simulink model "Homework4_P1"  (R2023b)
settings: Solver=FixedStepDiscrete  StartTime=0.0  StopTime=1  FixedStep=0.002  RelTol=1e-3  EnableMultiTasking=on
values from neighbouring files (symbols this model uses):
  Beta = [B_0 ; B_1 ; B_2 ; B_3]    [Homework4.m]
  phi = 45    [Homework4.m]
  psi = 60    [Homework4.m]
  theta = 30    [Homework4.m]
undefined symbols (not defined in the file or in its folder): a, alpha
settings Model: ExtModeTrigDuration=10000  Creator=jtmil  LastModifiedBy=jtmil
settings SolverCC: AlgebraicLoopSolver=TrustRegion  PositivePriorityOrder=on
settings DataIOCC: ReturnWorkspaceOutputs=off
settings OptimizationCC: LifeSpan=inf
settings DebuggingCC: UnconnectedInputMsg=warning  UnconnectedOutputMsg=warning  UnconnectedLineMsg=warning  ArithmeticOperatorsInVariantConditions=warning
settings ModelReferenceCC: EnableRefExpFcnMdlSchedulingChecks=on
settings SFSimCC: SimUseLocalCustomCode=off  CustomCodeUndefinedFunction=UseInterfaceOnly
settings RTWCC: Description=QUARC Win64 Target  SystemTargetFile=quarc_win64.tlc  TemplateMakefile=quarc_default_tmf  RTWUseLocalCustomCode=off
settings CodeAppCC: StateflowObjectComments=on
settings STFCustomTargetCC: TargetPreCompLibLocation=C:\PROGRA~3\QUARC\lib\2016a\win64\release  ConcurrentExecutionCompliant=on  GRTInterface=on  SystemTargetFile=quarc_win64.tlc
settings GRTTargetCC: TargetPreCompLibLocation=C:\PROGRA~3\QUARC\lib\2016a\win64\release  ParMdlRefBuildCompliant=off  CompOptLevelCompliant=off  CombineOutputUpdateFcns=off  MatFileLogging=off  CPPClassGenCompliant=off  GRTInterface=on  UseToolchainInfoCompliant=off  ExtMode=on  ExtModeMexFile=quarc_comm
settings ConfigComp: CovMetricSettings=dswe

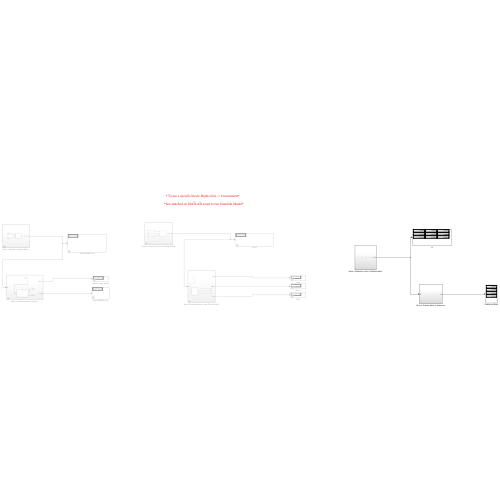
[thumbnail: Simulink's stored preview of the top-level diagram]
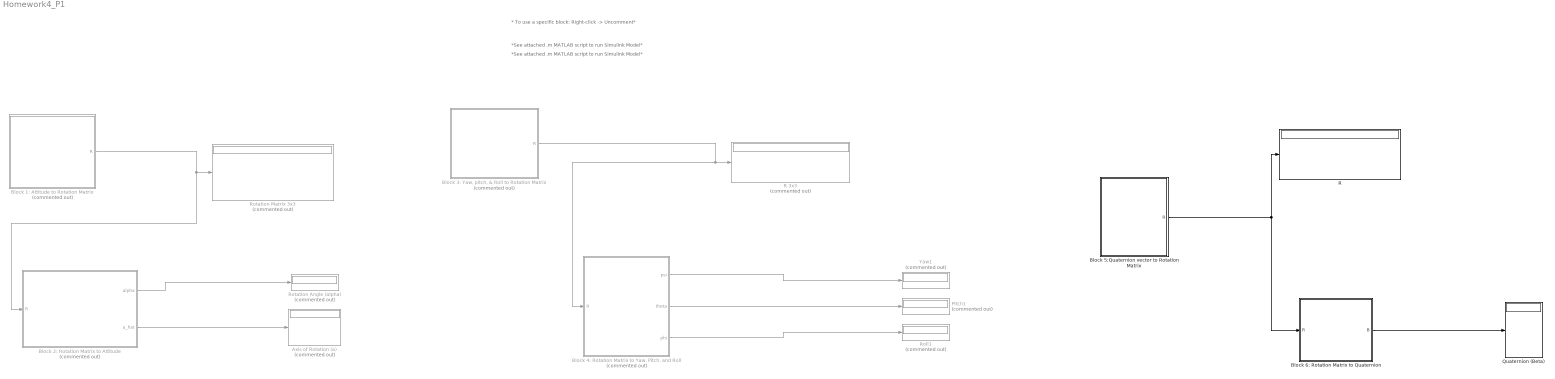
== system Homework4_P1 ==
  note: *See attached .m MATLAB script to run Simulink Model*
  note: * To use a specific block: Right-click -> Uncomment*
  note: *See attached .m MATLAB script to run Simulink Model*
  Axis of Rotation (a) : Display  Commented=on
  Block 1: Attitude to Rotation Matrix : Subsystem  Commented=on
  "Block 2: Rotation Matrix to Attitude " : Subsystem  Commented=on
  "Block 3: Yaw, pitch, & Roll to Rotation Matrix" : Subsystem  Commented=on
  "Block 4: Rotation Matrix to Yaw, Pitch, and Roll" : Subsystem  Commented=on
  Block 5:Quaternion vector to Rotation Matrix : Subsystem
  Block 6: Rotation Matrix to Quaternion : Subsystem
  Pitch1 : Display  Commented=on
  Quaternion (Beta) : Display
  R : Display
  R 3x3 : Display  Commented=on
  Roll1 : Display  Commented=on
  Rotation Angle (alpha) : Display  Commented=on
  Rotation Matrix 3x3 : Display  Commented=on
  Yaw1 : Display  Commented=on
  wires:
  Block 5:Quaternion vector to Rotation Matrix/1(R) -> Block 6: Rotation Matrix to Quaternion/1(R), R/1
  Block 6: Rotation Matrix to Quaternion/1(B) -> Quaternion (Beta)/1
  Block 1: Attitude to Rotation Matrix/1(R) -> "Block 2: Rotation Matrix to Attitude "/1(R), Rotation Matrix 3x3/1
  "Block 2: Rotation Matrix to Attitude "/1(alpha) -> Rotation Angle (alpha)/1
  "Block 2: Rotation Matrix to Attitude "/2(a_hat) -> Axis of Rotation (a)/1
  "Block 3: Yaw, pitch, & Roll to Rotation Matrix"/1(R) -> "Block 4: Rotation Matrix to Yaw, Pitch, and Roll"/1(R), R 3x3/1
  "Block 4: Rotation Matrix to Yaw, Pitch, and Roll"/1(psi) -> Yaw1/1
  "Block 4: Rotation Matrix to Yaw, Pitch, and Roll"/2(theta) -> Pitch1/1
  "Block 4: Rotation Matrix to Yaw, Pitch, and Roll"/3(phi) -> Roll1/1

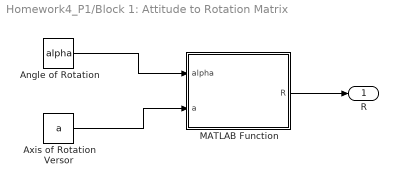
== system Homework4_P1/Block 1: Attitude to Rotation Matrix ==
  Angle of Rotation : Constant  Value=alpha
  Axis of Rotation Versor : Constant  Value=a
  MATLAB Function : MATLAB Function  TreatAsAtomicUnit=on
  R : Outport
  wires:
  Axis of Rotation Versor/1 -> MATLAB Function/2(a)
  Angle of Rotation/1 -> MATLAB Function/1(alpha)
  MATLAB Function/1(R) -> R/1

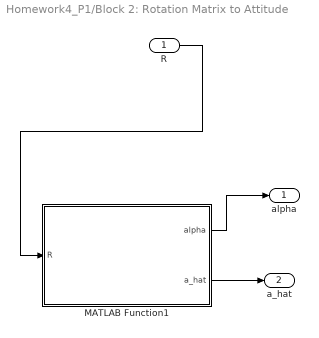
== system Homework4_P1/Block 2: Rotation Matrix to Attitude  ==
  R : Inport
  MATLAB Function1 : MATLAB Function  TreatAsAtomicUnit=on
  alpha : Outport
  a_hat : Outport  Port=2
  wires:
  MATLAB Function1/2(a_hat) -> a_hat/1
  R/1 -> MATLAB Function1/1(R)
  MATLAB Function1/1(alpha) -> alpha/1

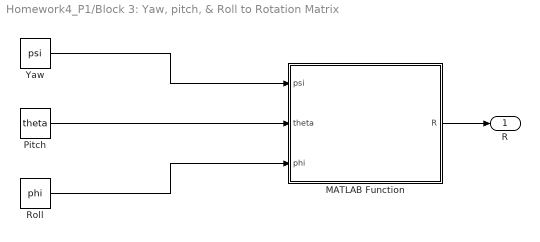
== system Homework4_P1/Block 3: Yaw, pitch, & Roll to Rotation Matrix ==
  MATLAB Function : MATLAB Function  TreatAsAtomicUnit=on
  Pitch : Constant  Value=theta
  Roll : Constant  Value=phi
  Yaw : Constant  Value=psi
  R : Outport
  wires:
  Pitch/1 -> MATLAB Function/2(theta)
  MATLAB Function/1(R) -> R/1
  Roll/1 -> MATLAB Function/3(phi)
  Yaw/1 -> MATLAB Function/1(psi)

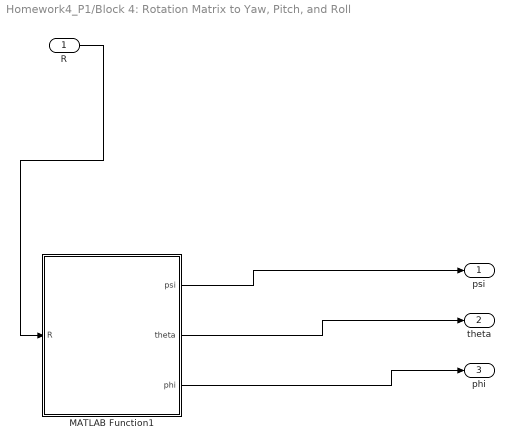
== system Homework4_P1/Block 4: Rotation Matrix to Yaw, Pitch, and Roll ==
  R : Inport
  MATLAB Function1 : MATLAB Function  TreatAsAtomicUnit=on
  psi : Outport
  theta : Outport  Port=2
  phi : Outport  Port=3
  wires:
  MATLAB Function1/1(psi) -> psi/1
  MATLAB Function1/3(phi) -> phi/1
  MATLAB Function1/2(theta) -> theta/1
  R/1 -> MATLAB Function1/1(R)

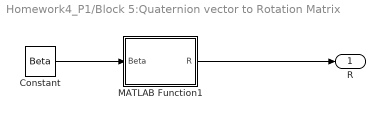
== system Homework4_P1/Block 5:Quaternion vector to Rotation Matrix ==
  Constant : Constant  Value=Beta
  MATLAB Function1 : MATLAB Function  TreatAsAtomicUnit=on
  R : Outport
  wires:
  Constant/1 -> MATLAB Function1/1(Beta)
  MATLAB Function1/1(R) -> R/1

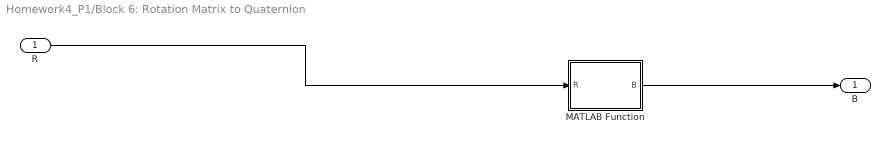
== system Homework4_P1/Block 6: Rotation Matrix to Quaternion ==
  R : Inport
  MATLAB Function : MATLAB Function  TreatAsAtomicUnit=on
  B : Outport
  wires:
  MATLAB Function/1(B) -> B/1
  R/1 -> MATLAB Function/1(R)

== matlab function Homework4_P1/Block 3: Yaw, pitch, & Roll to Rotation Matrix/MATLAB Function ==
  data: psi input; R output; theta input; phi input
function R  = fcn(psi,theta, phi)

R1 = [ 1 0 0  ; 0 cosd(phi) sind(phi) ; 0 -sind(phi) cosd(phi)];
R2 = [cosd(theta) 0 -sind(theta); 0 1 0; sind(theta) 0 cosd(theta)];
R3 = [ cosd(psi) sind(psi) 0 ; -sind(psi) cosd(psi) 0 ; 0 0 1];

R = R1*R2*R3

end

== matlab function Homework4_P1/Block 4: Rotation Matrix to Yaw, Pitch, and Roll/MATLAB Function1 ==
  data: R input; psi output; theta output; phi output
function [psi,theta,phi] = fcn(R)

phi = atan2d(R(1,2) , R(1,1)) % Yaw
theta = asind(-R(1,3))        % Pitch
psi = atan2d(R(2,3),R(3,3))   % Roll

end

== matlab function Homework4_P1/Block 1: Attitude to Rotation Matrix/MATLAB Function ==
  data: alpha input; R output; a input
function R  = fcn(alpha, a)

a_hat = a/norm(a);               % Normalize vector a
a_hat_transpose = a_hat';        % Transpose Vector a
a_skew_symmetric = [0 -a(3) a(2); a(3) 0 -a(1); -a(2) a(1) 0]; % Skew Symmetric Matrix of a
I = eye(3);                       % Identity Matrix

R = cosd(alpha)*I + (1-cosd(alpha))*(a_hat*a_hat_transpose) - sind(alpha)*a_skew_symmetric; % Euler's Formula



end

== matlab function Homework4_P1/Block 6: Rotation Matrix to Quaternion/MATLAB Function ==
  data: R input; B output
function B = fcn(R)

B_0_check = (1/4)*(1 + R(1,1) + R(2,2) + R(3,3));
B_1_check = (1/4)*(1 + R(1,1) - R(2,2) - R(3,3));
B_2_check = (1/4)*(1 + R(2,2) - R(1,1) - R(3,3));
B_3_check = (1/4)*(1 + R(3,3) - R(1,1) - R(2,2));

B_check = [B_0_check ; B_1_check ; B_2_check ; B_3_check];

B_max = max(B_check);

% Initialize variables to ensure they are defined
B_0 = 0;
B_1 = 0;
B_2 = 0;
B_3 = 0;

if B_max == B_0_check % B_0 is max
    B_0 = sqrt(B_0_check);
    B_1 = (1/(4*B_0))*(R(2,3) - R(3,2));
    B_2 = (1/(4*B_0))*(R(3,1) - R(1,3));
    B_3 = (1/(4*B_0))*(R(1,2) - R(2,1));
elseif B_max == B_1_check % B_1 is max
    B_1 = sqrt(B_1_check);
    B_0 = (1/(4*B_1))*(R(2,3) - R(3,2));
    B_2 = (1/(4*B_1))*(R(1,2) - R(2,1));
    B_3 = (1/(4*B_1))*(R(3,1) - R(1,3));
elseif B_max == B_2_check % B_2 is max
    B_2 = sqrt(B_2_check);
    B_0 = (1/(4*B_2))*(R(3,1) - R(1,3));
    B_1 = (1/(4*B_2))*(R(1,2) + R(2,1));
    B_3 = (1/(4*B_2))*(R(2,3) + R(3,2));
elseif B_max == B_3_check % B_3 is max
    B_3 = sqrt(B_3_check);
    B_0 = (1/(4*B_3))*(R(1,2) - R(2,1));
    B_1 = (1/(4*B_3))*(R(3,1) + R(1,3));
    B_2 = (1/(4*B_3))*(R(2,3) + R(3,2));
end

B = [B_0 ; B_1 ; B_2 ; B_3];

if any(B < 0)
    B = -1*B;
end

end

== matlab function Homework4_P1/Block 5:Quaternion vector to Rotation Matrix/MATLAB Function1 ==
  data: Beta input; R output
function R  = fcn(Beta)


R = [Beta(1)^2 + Beta(2)^2 - Beta(3)^2 - Beta(4)^2, 2*Beta(2)*Beta(3) + 2*Beta(1)*Beta(4), 2*Beta(2)*Beta(4) - 2*Beta(1)*Beta(3);
     2*Beta(2)*Beta(3) - 2*Beta(1)*Beta(4), Beta(1)^2 - Beta(2)^2 + Beta(3)^2 - Beta(4)^2, 2*Beta(3)*Beta(4) + 2*Beta(1)*Beta(2);
     2*Beta(2)*Beta(4) + 2*Beta(1)*Beta(3), 2*Beta(3)*Beta(4) - 2*Beta(1)*Beta(2), Beta(1)^2 - Beta(2)^2 - Beta(3)^2 + Beta(4)^2];



end

== matlab function Homework4_P1/Block 2: Rotation Matrix to Attitude /MATLAB Function1 ==
  data: R input; alpha output; a_hat output
function [alpha, a_hat] = fcn(R)

% Initialize alpha and a_hat
alpha = acosd((1/2)*(R(1,1) + R(2,2) + R(3,3) - 1));


a_hat = [1; 0; 0]; 

if alpha == 0  
    a_hat = [1; 0; 0];
elseif alpha == 180
    if R(1,1) ~= -1
        a_hat_x = abs(sqrt((R(1,1) + 1) / 2));
        a_hat = [a_hat_x; R(1,2) / (2 * a_hat_x); R(1,3) / (2 * a_hat_x)];
    elseif R(2,2) ~= -1
        a_hat_y = abs(sqrt((R(2,2) + 1) / 2));
        a_hat = [R(2,1) / (2 * a_hat_y); a_hat_y; R(2,3) / (2 * a_hat_y)];
    elseif R(3,3) ~= -1
        a_hat_z = abs(sqrt((R(3,3) + 1) / 2));
        a_hat = [R(3,1) / (2 * a_hat_z); R(3,2) / (2 * a_hat_z); a_hat_z];
    end
elseif alpha > 0 && alpha < 180
    a_hat = (1 / (2 * sind(alpha))) * [R(2,3) - R(3,2); R(3,1) - R(1,3); R(1,2) - R(2,1)];
end

end
